simulink model "two_property_PP_with_cocospec"  (R2015a)
settings: Solver=FixedStepDiscrete  StartTime=0.0  StopTime=10.0  RelTol=1e-3
model workspace (MAT data in the model file):
  already_pp = 1
settings Model: CovSFcnEnable=off  Creator=arnaud  LastModifiedBy=hbourbou
settings DataIOCC: SaveFormat=Structure  SignalLoggingSaveFormat=ModelDataLogs
settings OptimizationCC: ExpressionDepthLimit=2147483647
settings DebuggingCC: UnderspecifiedInitializationDetection=Classic  MergeDetectMultiDrivingBlocksExec=none  SolverPrmCheckMsg=warning  FcnCallInpInsideContextMsg=EnableAllAsWarning  StateNameClashWarn=warning
settings GRTTargetCC: CombineOutputUpdateFcns=off  GRTInterface=on

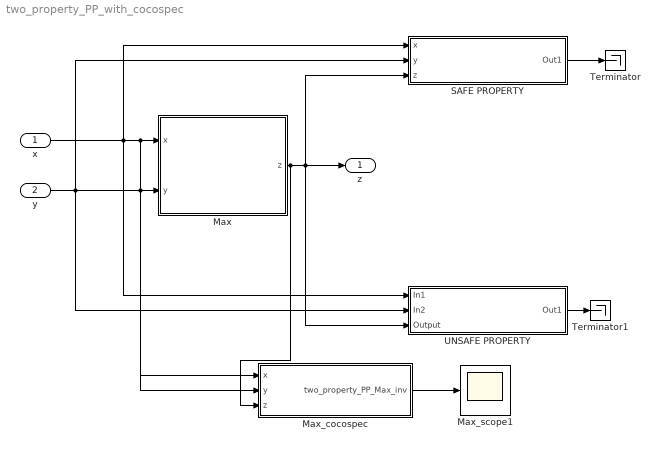
== system two_property_PP_with_cocospec ==
  x : Inport  OutDataTypeStr=int32
  y : Inport  Port=2  OutDataTypeStr=int32
  Max : Subsystem  TreatAsAtomicUnit=on
      settings: MinAlgLoopOccurrences=on
  Max_cocospec : Subsystem  mask(Observer){AnnotationType=assert, ObserverType=[]}
      mask prompts: AnnotationType "Type of annotation (pre/post...)"; ObserverType "Observer type"
      mask help:
      | Set an observer for the system.
      | The annotation type parameter sets the type of observer:
      | - requires : pre-condition
      | - ensures : post-condition
      | - assert : an assertion
      | - observer : the observer computes a special type of properties
      mask TypeOptions AnnotationType: ensures | requires | assert | observer
      mask Callback AnnotationType:
      | paramStr = get_param(gcb, 'MaskValues');
      | if strcmp(paramStr{1}(1),'o')
      | set_param(gcb,'MaskVisibilities',{'on';'on'});
      | paramStr{2} = 'ellipsoid';
      | set_param(gcb,'MaskValues',paramStr);
      | else
      | set_param(gcb,'MaskVisibilities',{'on';'off'});
      | end
      | clear paramStr;
      mask Callback ObserverType:
      | paramStr = get_param(gcb, 'MaskValues');
      | if strcmp(paramStr{1}(1),'o')
      | set_param(gcb,'MaskVisibilities',{'on';'on'});
      | paramStr{2} = 'ellipsoid';
      | set_param(gcb,'MaskValues',paramStr);
      | else
      | set_param(gcb,'MaskVisibilities',{'on';'off'});
      | end
      | clear paramStr;
      mask Display:
      | color('red')
      | text(0.5, 0.5, ['CoCoSpec: ''' get_param(gcb,'name') ''''], 'horizontalAlignment', 'center');
      | text(0.99, 0.03, '{\bf\fontsize{12}INVARIANT}', 'hor', 'right', 'ver', 'bottom', 'texmode', 'on');
  Max_scope1 : Scope
      settings: TimeRange=auto  MaxDataPoints=5000  SaveToWorkspace=off  SaveName=ScopeData  YMin=0.9  YMax=1.1  SampleTime=-1
  SAFE PROPERTY : Subsystem  TreatAsAtomicUnit=on  mask(Observer){AnnotationType=ensures, ObserverType=ellipsoid}
      mask prompts: AnnotationType "Type of annotation (pre/post...)"; ObserverType "Observer type"
      mask help:
      | Set an observer for the system.
      | The annotation type parameter sets the type of observer:
      | - requires : pre-condition
      | - ensures : post-condition
      | - assert : an assertion
      | - observer : the observer computes a special type of properties
      settings: MinAlgLoopOccurrences=on
      mask TypeOptions AnnotationType: ensures | requires | assert | observer
      mask Callback AnnotationType:
      | paramStr = get_param(gcb, 'MaskValues');
      | 
      | if strcmp(paramStr{1}(1),'o')
      |     set_param(gcb,'MaskVisibilities',{'on';'on'});
      |     paramStr{2} = 'ellipsoid';
      |     set_param(gcb,'MaskValues',paramStr);
      | else
      |     set_param(gcb,'MaskVisibilities',{'on';'off'});
      | end
      mask Callback ObserverType:
      | paramStr = get_param(gcb, 'MaskValues');
      | 
      | if strcmp(paramStr{1}(1),'observer')
      |     set_param(gcb,'MaskVisibilities',{'on';'on'});
      |     paramStr{2} = 'ellipsoid';
      |     set_param(gcb,'MaskValues',paramStr);
      | else
      |     set_param(gcb,'MaskVisibilities',{'on';'off'});
      | end
      mask Display:
      | color('black')
      | text(0.5, 0.5, ['Property: ''' get_param(gcb,'name') ''''], 'horizontalAlignment', 'center');
      | text(0.99, 0.03, '{\bf\fontsize{12}SAFE}', 'hor', 'right', 'ver', 'bottom', 'texmode', 'on');
  Terminator : Terminator
  Terminator1 : Terminator
  UNSAFE PROPERTY : Subsystem  TreatAsAtomicUnit=on  mask(Observer){AnnotationType=ensures, ObserverType=ellipsoid}
      mask prompts: AnnotationType "Type of annotation (pre/post...)"; ObserverType "Observer type"
      mask help:
      | Set an observer for the system.
      | The annotation type parameter sets the type of observer:
      | - requires : pre-condition
      | - ensures : post-condition
      | - assert : an assertion
      | - observer : the observer computes a special type of properties
      settings: MinAlgLoopOccurrences=on
      mask TypeOptions AnnotationType: ensures | requires | assert | observer
      mask Callback AnnotationType:
      | paramStr = get_param(gcb, 'MaskValues');
      | 
      | if strcmp(paramStr{1}(1),'o')
      |     set_param(gcb,'MaskVisibilities',{'on';'on'});
      |     paramStr{2} = 'ellipsoid';
      |     set_param(gcb,'MaskValues',paramStr);
      | else
      |     set_param(gcb,'MaskVisibilities',{'on';'off'});
      | end
      mask Callback ObserverType:
      | paramStr = get_param(gcb, 'MaskValues');
      | 
      | if strcmp(paramStr{1}(1),'observer')
      |     set_param(gcb,'MaskVisibilities',{'on';'on'});
      |     paramStr{2} = 'ellipsoid';
      |     set_param(gcb,'MaskValues',paramStr);
      | else
      |     set_param(gcb,'MaskVisibilities',{'on';'off'});
      | end
      mask Display:
      | color('black')
      | text(0.5, 0.5, ['Property: ''' get_param(gcb,'name') ''''], 'horizontalAlignment', 'center');
      | text(0.99, 0.03, '{\bf\fontsize{12}CEX}', 'hor', 'right', 'ver', 'bottom', 'texmode', 'on');
  z : Outport
  wires:
  x/1 -> Max_cocospec/1(x), Max/1(x), UNSAFE PROPERTY/1(In1), SAFE PROPERTY/1(x)
  y/1 -> Max_cocospec/2(y), Max/2(y), UNSAFE PROPERTY/2(In2), SAFE PROPERTY/2(y)
  SAFE PROPERTY/1(Out1) -> Terminator/1
  UNSAFE PROPERTY/1(Out1) -> Terminator1/1
  Max/1(z) -> SAFE PROPERTY/3(z), z/1, UNSAFE PROPERTY/3(Output), Max_cocospec/3(z)
  Max_cocospec/1(two_property_PP_Max_inv) -> Max_scope1/1

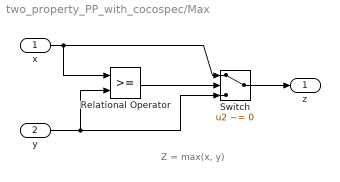
== system two_property_PP_with_cocospec/Max ==
  note: Z = max(x, y)
  x : Inport  OutDataTypeStr=int32
  y : Inport  Port=2  OutDataTypeStr=int32
  Relational Operator : RelationalOperator  OutDataTypeStr=boolean
  Switch : Switch  Criteria=u2 ~= 0
  z : Outport
  wires:
  Relational Operator/1 -> Switch/2
  Switch/1 -> z/1
  x/1 -> Relational Operator/1, Switch/1
  y/1 -> Switch/3, Relational Operator/2

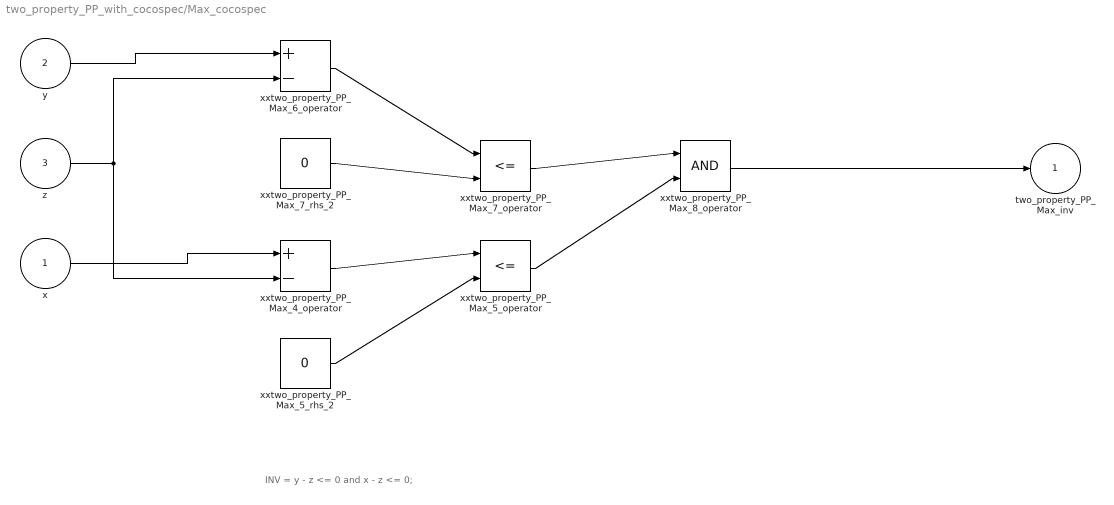
== system two_property_PP_with_cocospec/Max_cocospec ==
  note: INV = y - z <= 0 and x - z <= 0;
  x : Inport  OutDataTypeStr=int32
  y : Inport  Port=2  OutDataTypeStr=int32
  z : Inport  Port=3  OutDataTypeStr=int32
  xxtwo_property_PP_Max_4_operator : Sum  Inputs=+-  OutDataTypeStr=int32
  xxtwo_property_PP_Max_5_operator : RelationalOperator  Operator=<=  OutDataTypeStr=boolean
  xxtwo_property_PP_Max_5_rhs_2 : Constant  Value=0  OutDataTypeStr=int32
  xxtwo_property_PP_Max_6_operator : Sum  Inputs=+-  OutDataTypeStr=int32
  xxtwo_property_PP_Max_7_operator : RelationalOperator  Operator=<=  OutDataTypeStr=boolean
  xxtwo_property_PP_Max_7_rhs_2 : Constant  Value=0  OutDataTypeStr=int32
  xxtwo_property_PP_Max_8_operator : Logic  AllPortsSameDT=off  OutDataTypeStr=boolean
  two_property_PP_Max_inv : Outport
  wires:
  xxtwo_property_PP_Max_7_operator/1 -> xxtwo_property_PP_Max_8_operator/1
  xxtwo_property_PP_Max_5_rhs_2/1 -> xxtwo_property_PP_Max_5_operator/2
  z/1 -> xxtwo_property_PP_Max_4_operator/2, xxtwo_property_PP_Max_6_operator/2
  x/1 -> xxtwo_property_PP_Max_4_operator/1
  y/1 -> xxtwo_property_PP_Max_6_operator/1
  xxtwo_property_PP_Max_4_operator/1 -> xxtwo_property_PP_Max_5_operator/1
  xxtwo_property_PP_Max_7_rhs_2/1 -> xxtwo_property_PP_Max_7_operator/2
  xxtwo_property_PP_Max_6_operator/1 -> xxtwo_property_PP_Max_7_operator/1
  xxtwo_property_PP_Max_5_operator/1 -> xxtwo_property_PP_Max_8_operator/2
  xxtwo_property_PP_Max_8_operator/1 -> two_property_PP_Max_inv/1

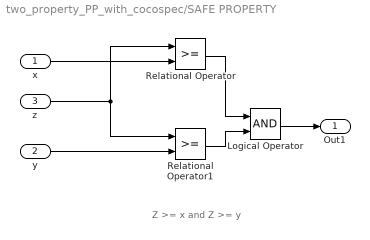
== system two_property_PP_with_cocospec/SAFE PROPERTY ==
  note: Z >= x and Z >= y
  x : Inport  OutDataTypeStr=int32
  y : Inport  Port=2  OutDataTypeStr=int32
  z : Inport  Port=3  OutDataTypeStr=int32
  Logical Operator : Logic  AllPortsSameDT=off  OutDataTypeStr=boolean
  Relational Operator : RelationalOperator  OutDataTypeStr=boolean
  Relational Operator1 : RelationalOperator  OutDataTypeStr=boolean
  Out1 : Outport
  wires:
  Relational Operator/1 -> Logical Operator/1
  Relational Operator1/1 -> Logical Operator/2
  Logical Operator/1 -> Out1/1
  z/1 -> Relational Operator/1, Relational Operator1/1
  x/1 -> Relational Operator/2
  y/1 -> Relational Operator1/2

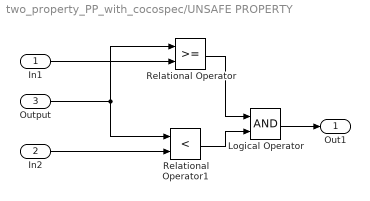
== system two_property_PP_with_cocospec/UNSAFE PROPERTY ==
  In1 : Inport  OutDataTypeStr=int32
  In2 : Inport  Port=2  OutDataTypeStr=int32
  Output : Inport  Port=3  OutDataTypeStr=int32
  Logical Operator : Logic  AllPortsSameDT=off  OutDataTypeStr=boolean
  Relational Operator : RelationalOperator  OutDataTypeStr=boolean
  Relational Operator1 : RelationalOperator  Operator=<  OutDataTypeStr=boolean
  Out1 : Outport
  wires:
  Relational Operator/1 -> Logical Operator/1
  Relational Operator1/1 -> Logical Operator/2
  Logical Operator/1 -> Out1/1
  Output/1 -> Relational Operator/1, Relational Operator1/1
  In1/1 -> Relational Operator/2
  In2/1 -> Relational Operator1/2
